simulink model "Tachometer_Q4"  (R2015b)
settings: Solver=FixedStepDiscrete  StartTime=0.0  StopTime=inf  FixedStep=0.005  RelTol=1e-3
undefined symbols (not defined in the file): DiscIntNeverNeededParam, fdesignblkfcn, gcbh, HIL, qc_get_step_size
libraries: quarc_library x4, dsparch4 x1
settings Model: SimulationMode=external  ExtModeTrigDuration=5000  Creator=Admin  LastModifiedBy=Admin
settings SolverCC: PositivePriorityOrder=on
settings DataIOCC: SaveFormat=Array  SignalLoggingSaveFormat=ModelDataLogs
settings OptimizationCC: ExpressionDepthLimit=2147483647
settings DebuggingCC: UnderspecifiedInitializationDetection=Classic  MergeDetectMultiDrivingBlocksExec=none  SolverPrmCheckMsg=warning  FcnCallInpInsideContextMsg=UseLocalSettings  StateNameClashWarn=warning
settings HardwareCC: ProdBitPerPointer=32  ProdLargestAtomicFloat=None  ProdIntDivRoundTo=Undefined  ProdEndianess=Unspecified  ProdWordSize=32  ProdHWDeviceType=32-bit Generic
settings RTWCC: SystemTargetFile=quarc_win64.tlc  TemplateMakefile=quarc_default_tmf  Description=QUARC Win64 Target
settings STFCustomTargetCC: GeneratePreprocessorConditionals=Use local settings  CPPClassGenCompliant=off
settings GRTTargetCC: ParMdlRefBuildCompliant=off  CompOptLevelCompliant=off  CombineOutputUpdateFcns=off  MatFileLogging=off  CPPClassGenCompliant=off  GRTInterface=on  UseToolchainInfoCompliant=off  ExtMode=on  ExtModeMexFile=quarc_comm
settings ConfigComp: CovModelRefEnable=Off

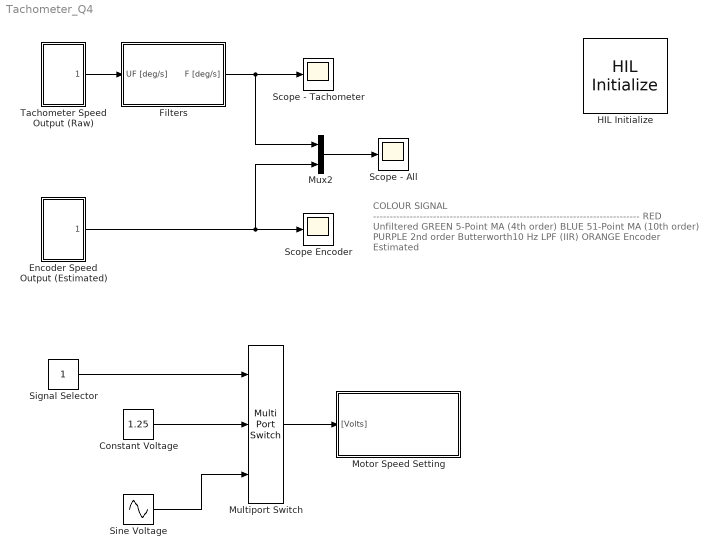
== system Tachometer_Q4 ==
  note: COLOUR SIGNAL
      | --------------------------------------------------------------------------------
      | RED Unfiltered
      | GREEN 5-Point MA (4th order)
      | BLUE 51-Point MA (10th order)
      | PURPLE 2nd order Butterworth10 Hz LPF (IIR)
      | ORANGE Encoder Estimated
  Constant Voltage : Constant  Value=1.25
  Encoder Speed Output (Estimated) : Subsystem
  Filters : Subsystem
  HIL Initialize : quarc_library/Data Acquisition/Generic/Configuration/HIL Initialize  object_name=HIL-1  board_type=q4  board_number=0  board_options=""  exclusive=off  active=off  hardware_clocks=[0:1]  clock_modes=[0 0]  initial_clock_frequencies=[]  set_clock_params_at_start=on  set_clock_params_at_switch_in=off  set_clock_frequencies_at_start=off  set_clock_frequencies_at_switch_in=off  analog_input_channels=[0:3]  analog_input_maximums=10  analog_input_minimums=-10  set_analog_input_params_at_start=off  set_analog_input_params_at_switch_in=off  analog_output_channels=[0:3]  analog_output_maximums=[10]  analog_output_minimums=[-10]  initial_analog_outputs=[0]  final_analog_outputs=[0]  watchdog_analog_outputs=0  set_analog_output_params_at_start=on  set_analog_output_params_at_switch_in=off  set_analog_outputs_at_start=on  set_analog_outputs_at_switch_in=off  set_analog_outputs_at_terminate=on  set_analog_outputs_at_switch_out=off  set_analog_outputs_on_watchdog=off  digital_input_channels=[]  digital_output_channels=[]  digital_output_configuration=[]  initial_digital_outputs=[1]  final_digital_outputs=[1]  watchdog_digital_outputs=[2]  set_digital_output_params_at_start=off  set_digital_output_params_at_switch_in=off  set_digital_outputs_at_start=on  set_digital_outputs_at_switch_in=off  set_digital_outputs_at_terminate=on  set_digital_outputs_at_switch_out=off  set_digital_outputs_on_watchdog=off  encoder_channels=[0:3]  quadrature=[4]  encoder_filter_frequency=(1/60e-9)/1  initial_encoder_counts=[0]  set_encoder_params_at_start=on  set_encoder_params_at_switch_in=off  set_encoder_counts_at_start=on  set_encoder_counts_at_switch_in=off  pwm_channels=[]  pwm_modes=[0]  pwm_frequency=(1/60e-9)/1024  pwm_configuration=[]  pwm_alignment=[]  pwm_polarity=[]  pwm_leading_deadband=[]  pwm_trailing_deadband=[]  initial_pwm_outputs=[0]  final_pwm_outputs=[0]  watchdog_pwm_outputs=[]  set_pwm_params_at_start=on  set_pwm_params_at_switch_in=off  set_pwm_outputs_at_start=on  set_pwm_outputs_at_switch_in=off  set_pwm_outputs_at_terminate=on  set_pwm_outputs_at_switch_out=off  set_pwm_outputs_on_watchdog=off  other_output_channels=[]  initial_other_outputs=[]  final_other_outputs=[]  watchdog_other_outputs=[]  set_other_outputs_at_start=off  set_other_outputs_at_switch_in=off  set_other_outputs_at_terminate=off  set_other_outputs_at_switch_out=off  set_other_outputs_on_watchdog=off
  Motor Speed Setting : Subsystem
  Multiport Switch : MultiPortSwitch  Inputs=2
  Mux2 : Mux  Inputs=2
  Scope Encoder : Scope
  "Scope - All " : Scope
  Scope - Tachometer : Scope
  Signal Selector : Constant
  Sine Voltage : Sin  Amplitude=.25  Bias=1  Frequency=2*pi  SampleTime=qc_get_step_size
  Tachometer Speed Output (Raw) : Subsystem
  wires:
  Filters/1(F [deg/s]) -> Scope - Tachometer/1, Mux2/1
  Encoder Speed Output (Estimated)/1("[deg/s]") -> Scope Encoder/1, Mux2/2
  Mux2/1 -> "Scope - All "/1
  Tachometer Speed Output (Raw)/1("[deg/s]") -> Filters/1(UF [deg/s])
  Signal Selector/1 -> Multiport Switch/1
  Multiport Switch/1 -> Motor Speed Setting/1("[Volts]")
  Sine Voltage/1 -> Multiport Switch/3
  Constant Voltage/1 -> Multiport Switch/2

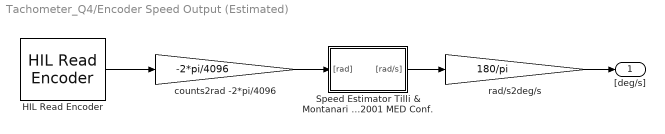
== system Tachometer_Q4/Encoder Speed Output (Estimated) ==
  HIL Read Encoder : quarc_library/Data Acquisition/Generic/Immediate I//O/HIL Read Encoder  object_name=HIL-1  channels=0  sample_time=qc_get_step_size  active=on  vector_output=off  data_type_mode=Inherit via back propagation  data_type=double
  Speed Estimator Tilli & Montanari 2001 MED Conf. : Subsystem
  counts2rad -2*pi/4096 : Gain  Gain=-2*pi/4096
  rad/s2deg/s : Gain  Gain=180/pi
  "[deg/s]" : Outport
  wires:
  HIL Read Encoder/1 -> counts2rad -2*pi/4096/1
  counts2rad -2*pi/4096/1 -> Speed Estimator Tilli & Montanari 2001 MED Conf./1("[rad]")
  Speed Estimator Tilli & Montanari 2001 MED Conf./1("[rad/s]") -> rad/s2deg/s/1
  rad/s2deg/s/1 -> "[deg/s]"/1

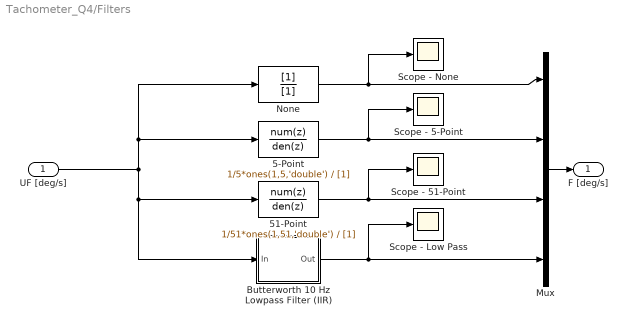
== system Tachometer_Q4/Filters ==
  UF [deg/s] : Inport
  5-Point : DiscreteFilter  Numerator=1/5*ones(1,5,'double')  Denominator=[1]
  51-Point : DiscreteFilter  Numerator=1/51*ones(1,51,'double')  Denominator=[1]
  Butterworth 10 Hz Lowpass Filter (IIR) : Subsystem  DialogController=fdesignblkfcn  InitFcn=fdesignblkfcn(gcbh, {'InitFcn'});  mask(Lowpass Filter){}
      mask help: Design a lowpass filter
      settings: CopyFcn=fdesignblkfcn(gcbh, {'CopyFcn'});
      mask Help: helpview(mapfilelocation('dsp'), 'dsplowpassfilter');
      mask Display: disp('Lowpass')
  Mux : Mux
  None : DiscreteFilter  Denominator=[1]
  Scope - 5-Point : Scope
  Scope - 51-Point : Scope
  Scope - Low Pass : Scope
  Scope - None : Scope
  F [deg/s] : Outport
  wires:
  Butterworth 10 Hz Lowpass Filter (IIR)/1(Out) -> Mux/4, Scope - Low Pass/1
  51-Point/1 -> Mux/3, Scope - 51-Point/1
  5-Point/1 -> Mux/2, Scope - 5-Point/1
  None/1 -> Mux/1, Scope - None/1
  UF [deg/s]/1 -> 51-Point/1, Butterworth 10 Hz Lowpass Filter (IIR)/1(In), None/1, 5-Point/1
  Mux/1 -> F [deg/s]/1

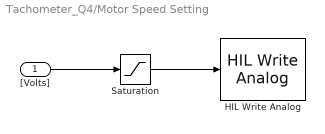
== system Tachometer_Q4/Motor Speed Setting ==
  "[Volts]" : Inport
  HIL Write Analog : quarc_library/Data Acquisition/Generic/Immediate I//O/HIL Write Analog  object_name=HIL-1  channels=0  sample_time=qc_get_step_size  active=off  vector_input=off
  Saturation : Saturate  UpperLimit=3  LowerLimit=-3
  wires:
  Saturation/1 -> HIL Write Analog/1
  "[Volts]"/1 -> Saturation/1

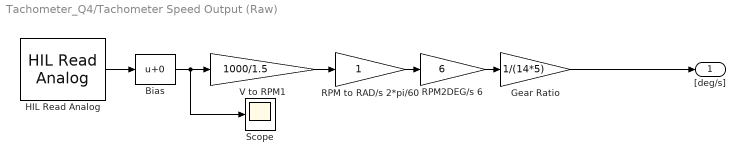
== system Tachometer_Q4/Tachometer Speed Output (Raw) ==
  Bias : Bias
  Gear Ratio : Gain  Gain=1/(14*5)
  HIL Read Analog : quarc_library/Data Acquisition/Generic/Immediate I//O/HIL Read Analog  object_name=HIL-1  channels=0  sample_time=qc_get_step_size  active=on  vector_output=off
  RPM to RAD/s 2*pi/60 : Gain
  RPM2DEG/s 6 : Gain  Gain=6
  Scope : Scope
  V to RPM1 : Gain  Gain=1000/1.5
  "[deg/s]" : Outport
  wires:
  Bias/1 -> Scope/1, V to RPM1/1
  Gear Ratio/1 -> "[deg/s]"/1
  RPM2DEG/s 6/1 -> Gear Ratio/1
  RPM to RAD/s 2*pi/60/1 -> RPM2DEG/s 6/1
  V to RPM1/1 -> RPM to RAD/s 2*pi/60/1
  HIL Read Analog/1 -> Bias/1

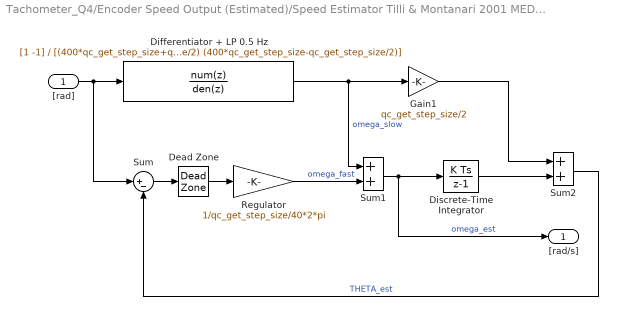
== system Tachometer_Q4/Encoder Speed Output (Estimated)/Speed Estimator Tilli & Montanari 2001 MED Conf. ==
  "[rad]" : Inport
  Dead Zone : DeadZone  LowerValue=-2*pi/4096  UpperValue=2*pi/4096  SaturateOnIntegerOverflow=on
  Differentiator + LP 0.5 Hz : DiscreteTransferFcn  Numerator=[1 -1]  Denominator=[(400*qc_get_step_size+qc_get_step_size/2) (400*qc_get_step_size-qc_get_step_size/2)]
  Discrete-Time Integrator : DiscreteIntegrator  SampleTime=-1  ICPrevOutput=DiscIntNeverNeededParam  ICPrevScaledInput=DiscIntNeverNeededParam
  Gain1 : Gain  Gain=qc_get_step_size/2
  Regulator : Gain  Gain=1/qc_get_step_size/40*2*pi
  Sum : Sum  Inputs=|+-
  Sum1 : Sum
  Sum2 : Sum
  "[rad/s]" : Outport
  wires:
  "[rad]"/1 -> Sum/1, Differentiator + LP 0.5 Hz/1
  Sum/1 -> Dead Zone/1
  Dead Zone/1 -> Regulator/1
  Regulator/1 -> Sum1/2  "omega_fast"
  Differentiator + LP 0.5 Hz/1 -> Sum1/1, Gain1/1  "omega_slow"
  Sum1/1 -> Discrete-Time Integrator/1, "[rad/s]"/1  "omega_est"
  Discrete-Time Integrator/1 -> Sum2/2
  Gain1/1 -> Sum2/1
  Sum2/1 -> Sum/2  "THETA_est"

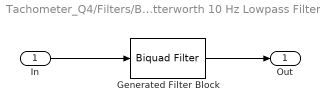
== system Tachometer_Q4/Filters/Butterworth 10 Hz Lowpass Filter (IIR) ==
  In : Inport
  Generated Filter Block : dsparch4/Biquad Filter  Tag=BlockMethodSubSystem  IIRFiltStruct=Direct form II  CoeffSource=Specify via dialog  BiQuadCoeffs=[0.250078647993701 0.500157295987402 0.250078647993701 1 -1.5610180758007179 0.64135153805756318]  a0Flag=Warning  IC=0  ICnum=0  ICden=0  InputProcessing=Columns as channels (frame based)  denAccumFracLength=30  denProdOutputFracLength=30  secondMemoryFracLength=15  roundingMode=Floor  overflowMode=off  ScaleValues=[0.080308197942261336;1]  optimizeScaleValues=off  ScaleValueMode=Specify via input port (g)  scaleValueFracLength=14  FilterSource=Specify via dialog  FilterObject=BQF
  Out : Outport
  wires:
  In/1 -> Generated Filter Block/1
  Generated Filter Block/1 -> Out/1
